simulink library "BMSLib"  (R2018b)
settings: Solver=VariableStepAuto  StartTime=0.0  StopTime=10.0  RelTol=1e-3
libraries: simulink_extras x1, simulink x1
settings Model: Creator=Santosh  LastModifiedBy=Santosh

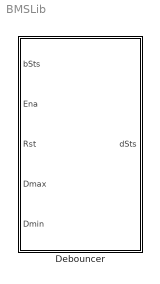
== system BMSLib ==
  Debouncer : Subsystem  mask(Debouncer){}
      mask help:
      | Debouncer IO
      | bSts : Fault flag or signal to be debounced (Bool)
      | Ena: Enables debouncer counting operation (Bool)
      | Rst: Resets the dounce counter and also the output to 0 (Bool)
      | Dmax: Max count at which the dSts is set (Int)
      | Dmin: Min count at which dSts is reset (Int)
      | dSts: Debounced output of bSts. (Bool)

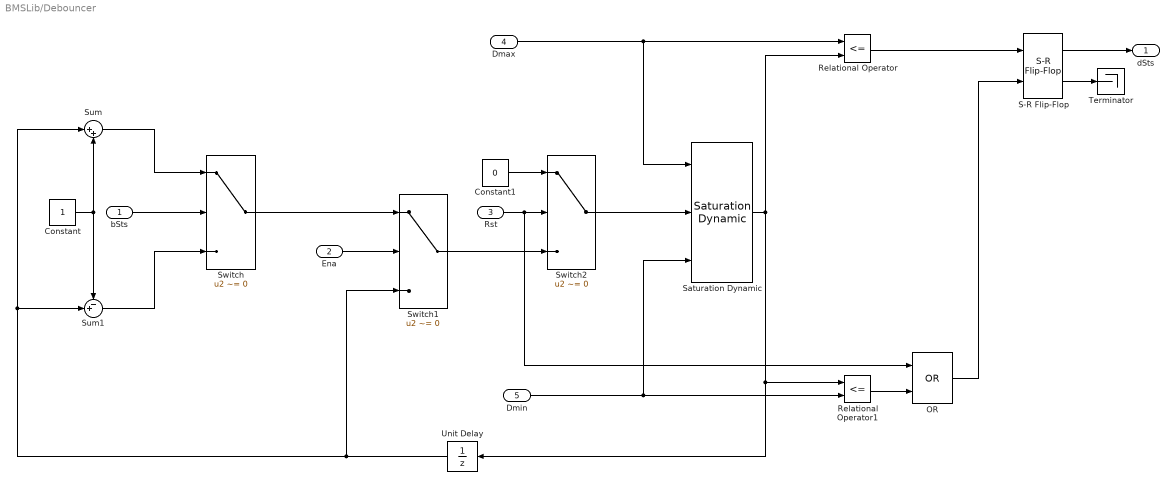
== system BMSLib/Debouncer ==
  bSts : Inport
  Ena : Inport  Port=2
  Rst : Inport  Port=3
  Dmax : Inport  Port=4
  Dmin : Inport  Port=5
  Constant : Constant
  Constant1 : Constant  Value=0
  OR : Logic  Operator=OR  IconShape=distinctive  AllPortsSameDT=off  OutDataTypeStr=boolean
  Relational Operator : RelationalOperator  Operator=<=  OutDataTypeStr=boolean  RndMeth=Simplest
  Relational Operator1 : RelationalOperator  Operator=<=  OutDataTypeStr=boolean  RndMeth=Simplest
  S-R Flip-Flop : simulink_extras/Flip Flops/S-R Flip-Flop  initial_condition=0
  Saturation Dynamic : simulink/Discontinuities/Saturation Dynamic  OutMin=[]  OutMax=[]  OutDataTypeStr=Inherit: Same as second input  OutDataType=fixdt(1, 16)  OutScaling=2^-10  DoSatur=off
  Sum : Sum  Inputs=|++
  Sum1 : Sum  Inputs=-+|
  Switch : Switch  Criteria=u2 ~= 0
  Switch1 : Switch  Criteria=u2 ~= 0
  Switch2 : Switch  Criteria=u2 ~= 0
  Terminator : Terminator
  Unit Delay : UnitDelay  SampleTime=-1
  dSts : Outport
  wires:
  Switch2/1 -> Saturation Dynamic/2
  Constant/1 -> Sum1/1, Sum/2
  Dmin/1 -> Relational Operator1/2, Saturation Dynamic/3
  S-R Flip-Flop/2 -> Terminator/1
  Unit Delay/1 -> Switch1/3, Sum/1, Sum1/2
  S-R Flip-Flop/1 -> dSts/1
  Constant1/1 -> Switch2/1
  Sum/1 -> Switch/1
  Saturation Dynamic/1 -> Relational Operator1/1, Unit Delay/1, Relational Operator/2
  Dmax/1 -> Saturation Dynamic/1, Relational Operator/1
  Rst/1 -> OR/1, Switch2/2
  Ena/1 -> Switch1/2
  Sum1/1 -> Switch/3
  Switch/1 -> Switch1/1
  Switch1/1 -> Switch2/3
  bSts/1 -> Switch/2
  Relational Operator/1 -> S-R Flip-Flop/1
  OR/1 -> S-R Flip-Flop/2
  Relational Operator1/1 -> OR/2
